simulink model "exampleWeather2WDB"  (Simulink 7.6)
settings: Solver=ode45  StartTime=0.0  StopTime=10.0  RelTol=1e-3
settings Model: Creator=drhf  LastModifiedBy=awohlfei
settings CodeAppCC: CustomSymbolStrType=$N$R$M_T

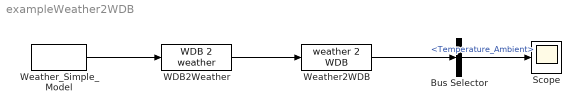
== system exampleWeather2WDB ==
  Bus Selector : BusSelector  OutputSignals=Temperature_Ambient
  Scope : Scope
  WDB2Weather : Reference  SystemSampleTime=-1
  Weather2WDB : Reference  SystemSampleTime=-1
  Weather_Simple_Model : Reference  SystemSampleTime=-1  lat=60  Ibn=900  Idg=100  tamb=5  deltaTsky=-6  rh=50  precip="10e-3/24/3600           % 10 mm in 24 h"  cloud=0.125  p=1013e2  vw=1  wdir=270
  wires:
  Weather_Simple_Model/1 -> WDB2Weather/1
  WDB2Weather/1 -> Weather2WDB/1
  Weather2WDB/1 -> Bus Selector/1
  Bus Selector/1 -> Scope/1  "<Temperature_Ambient>"
